simulink model "Bioreactor_for_olderversion_1_"  (R2025a)
settings: Solver=VariableStepAuto  StartTime=0.0  StopTime=2500  RelTol=1e-3
libraries: slpidlib x1, simulink x1
settings Model: Creator=a  LastModifiedBy=sayed
settings OptimizationCC: BlockReduction=off  DefaultParameterBehavior=Inlined  BufferReuse=off

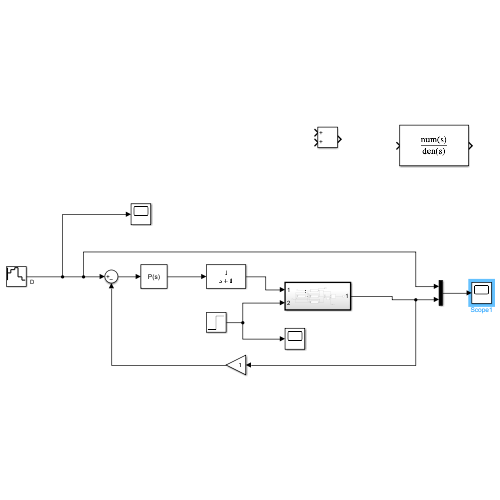
[thumbnail: Simulink's stored preview of the top-level diagram]
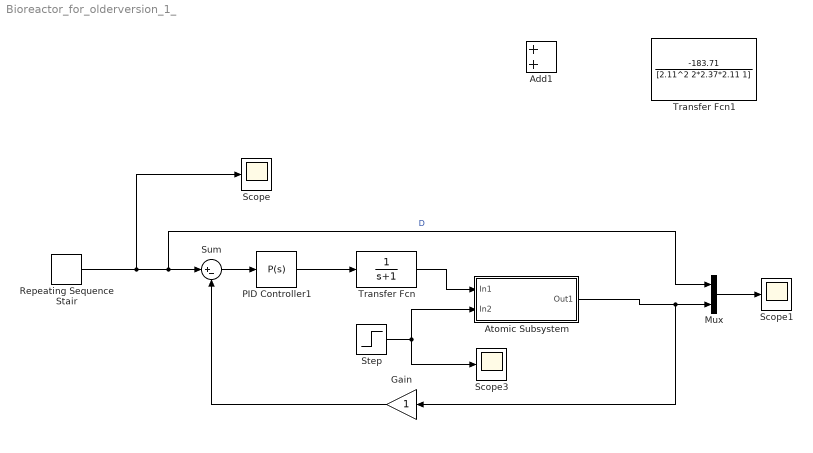
== system Bioreactor_for_olderversion_1_ ==
  Add1 : Sum
  Atomic Subsystem : Subsystem  TreatAsAtomicUnit=on
  Gain : Gain
  Mux : Mux  Inputs=2
  PID Controller1 : slpidlib/PID Controller  Controller=P  Form=Ideal  TimeDomain=Continuous-time  UseExternalTs=off  SampleTime=-1  IntegratorMethod=Forward Euler  FilterMethod=Forward Euler  ControllerParametersSource=internal  P=-0.0321  I=1/0.0992  UseKiTs=off  D=0.023  UseExternalDerivativeSource=off  N=100  UseFilter=on  TunerSelectOption=Transfer Function Based (PID Tuner App)  InitialConditionSource=internal  InitialConditionForIntegrator=0  InitialConditionForFilter=0  DifferentiatorICPrevScaledInput=0  ExternalReset=none  TrackingMode=off  Kt=1  LimitOutput=off  SatLimitsSource=internal  UpperSaturationLimit=inf  LowerSaturationLimit=-inf  LinearizeAsGain=on  AntiWindupMode=none  Kb=1  LimitIntegrator=off  UpperIntegratorSaturationLimit=inf  LowerIntegratorSaturationLimit=-inf  POutMin=[]  POutMax=[]  IOutMin=[]  IOutMax=[]  DOutMin=[]  DOutMax=[]  NOutMin=[]  NOutMax=[]  SumOutMin=[]  SumOutMax=[]  SaturationOutMin=[]  SaturationOutMax=[]  PParamMin=[]  PParamMax=[]  IParamMin=[]  IParamMax=[]  DParamMin=[]  DParamMax=[]  NParamMin=[]  NParamMax=[]  KbParamMin=[]  KbParamMax=[]  KtParamMin=[]  KtParamMax=[]  KbOutMin=[]  KbOutMax=[]  KtOutMin=[]  KtOutMax=[]  IntegratorOutMin=[]  IntegratorOutMax=[]  FilterOutMin=[]  FilterOutMax=[]  SumI1OutMin=[]  SumI1OutMax=[]  SumI2OutMin=[]  SumI2OutMax=[]  SumI3OutMin=[]  SumI3OutMax=[]  SumI4OutMin=[]  SumI4OutMax=[]  SumDOutMin=[]  SumDOutMax=[]  DifferentiatorOutMin=[]  DifferentiatorOutMax=[]  FilterDiffOutCoefMin=[]  FilterDiffOutCoefMax=[]  ReciprocalOutMin=[]  ReciprocalOutMax=[]  SumDenOutMin=[]  SumDenOutMax=[]  SumNumOutMin=[]  SumNumOutMax=[]  DivideOutMin=[]  DivideOutMax=[]  UdiffTsProdOutMin=[]  UdiffTsProdOutMax=[]  NTsProdOutMin=[]  NTsProdOutMax=[]  UintegralTsProdOutMin=[]  UintegralTsProdOutMax=[]  UngainTsProdOutMin=[]  UngainTsProdOutMax=[]  ClampingZeroOutDataTypeStr=Inherit: Inherit via back propagation  ClampingZeroOutMin=[]  ClampingZeroOutMax=[]  FilterDenConstantOutDataTypeStr=Inherit: Inherit via back propagation  FilterDenConstantOutMin=[]  FilterDenConstantOutMax=[]  PCopyOutDataTypeStr=Inherit: Inherit via back propagation  PCopyOutMin=[]  PCopyOutMax=[]  NCopyOutDataTypeStr=Inherit: Inherit via back propagation  NCopyOutMin=[]  NCopyOutMax=[]  IntegratorContinuousStateAttributes=''  IntegratorStateMustResolveToSignalObject=off  IntegratorRTWStateStorageClass=Auto  FilterContinuousStateAttributes=''  FilterStateMustResolveToSignalObject=off  FilterRTWStateStorageClass=Auto  ParallelPVariant=InternalParameters  IdealPVariant=Disabled  IVariant=Disabled  DVariant=Disabled  IntegratorVariant=Disabled  SatVariant=Disabled  AWVariant=Disabled  PCopyVariant=Disabled  TRVariant=Disabled  FdbkBlocksVariant=Forward  IdealPFdbkVariant=Disabled  SatFdbkVariant=Disabled  DerivativeFilterVariant=Disabled  NVariant=Disabled  NCopyVariant=Disabled_SignalSpec  FilterICVariant=Disabled  IntegratorICVariant=Disabled  ExternalResetVariant=Disabled  TRSumVariant=Passthrough  SumFdbkVariant=Disabled  SumVariant=Passthrough_P  TsampFilterVariant=InternalTs  TsampNgainVariant=Passthrough  TsampIntegralVariant=Disabled_SignalSpec  ExternalSaturationOutDataTypeStr=Inherit: Same as second input  DerivativeSourceVariant=Disabled  PreIntVariant=InternalPreInt
  Repeating Sequence Stair : simulink/Sources/Repeating Sequence Stair  OutValues=[2.6855 2.9 3 2.5 2.3 ].'  tsamp=500  OutMin=[]  OutMax=[]  OutDataTypeStr=double  OutputDataTypeScalingMode=double  OutDataType=fixdt(0,8)  ConRadixGroup=Best Precision: Vector-wise  OutScaling=2^-12
  Scope : Scope
      settings: ActiveDisplayYMinimum=-1  ActiveDisplayYMaximum=1
  Scope1 : Scope
      settings: ActiveDisplayYMinimum=-3.1572708705408776  ActiveDisplayYMaximum=29.415437834867905
  Scope3 : Scope
      settings: ActiveDisplayYMinimum=-1  ActiveDisplayYMaximum=1  DataLoggingVariableName=ScopeData9
  Step : Step  After=19.999  SampleTime=0
  Sum : Sum  Inputs=|+-
  Transfer Fcn : TransferFcn  Denominator=[1 1]
  Transfer Fcn1 : TransferFcn  Numerator=[-183.71]  Denominator=[2.11^2 2*2.37*2.11 1]
  wires:
  Repeating Sequence Stair/1 -> Mux/1, Sum/1, Scope/1  "D"
  Mux/1 -> Scope1/1
  Sum/1 -> PID Controller1/1
  PID Controller1/1 -> Transfer Fcn/1
  Transfer Fcn/1 -> Atomic Subsystem/1(In1)
  Gain/1 -> Sum/2
  Step/1 -> Scope3/1, Atomic Subsystem/2(In2)
  Atomic Subsystem/1(Out1) -> Gain/1, Mux/2

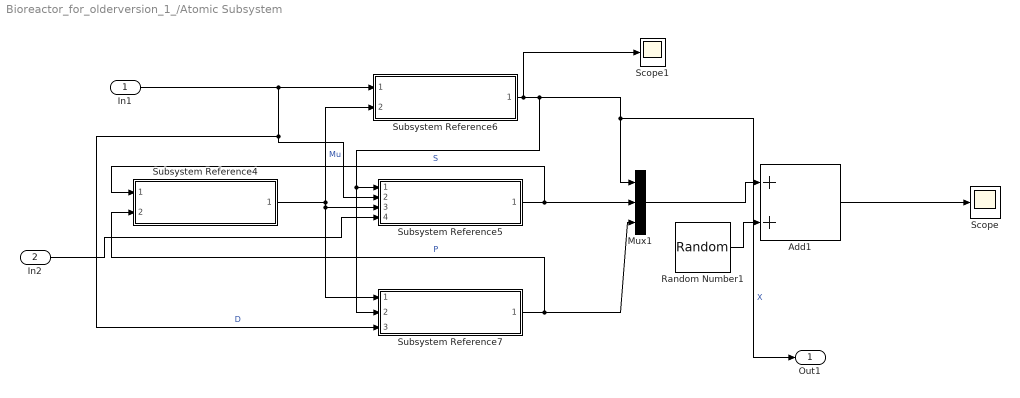
== system Bioreactor_for_olderversion_1_/Atomic Subsystem ==
  In1 : Inport
  In2 : Inport  Port=2
  Add1 : Sum
  Mux1 : Mux  Inputs=3
  Random Number1 : RandomNumber  Variance=0.01  SampleTime=0.1
  Scope : Scope
      settings: ActiveDisplayYMinimum=-9798.9196176080059  ActiveDisplayYMaximum=28688.615167165182  DataLoggingVariableName=ScopeData6
  Scope1 : Scope
      settings: ActiveDisplayYMinimum=-1  ActiveDisplayYMaximum=1  DataLoggingVariableName=ScopeData7
  Subsystem Reference4 : Subsystem  ReferencedSubsystem=Mu_SP_oldversion
  Subsystem Reference5 : Subsystem  ReferencedSubsystem=Substrate_oldVersion
  Subsystem Reference6 : Subsystem  ReferencedSubsystem=Biomass_X_oldversion
  Subsystem Reference7 : Subsystem  ReferencedSubsystem=Product_P_oldversion
  Out1 : Outport
  wires:
  Subsystem Reference6/1 -> Scope1/1, Out1/1, Mux1/1, Subsystem Reference7/2, Subsystem Reference5/1  "X"
  Random Number1/1 -> Add1/2
  Subsystem Reference7/1 -> Subsystem Reference4/2, Mux1/3  "P"
  Mux1/1 -> Add1/1
  Subsystem Reference5/1 -> Mux1/2, Subsystem Reference4/1  "S"
  Subsystem Reference4/1 -> Subsystem Reference7/1, Subsystem Reference5/3, Subsystem Reference6/2  "Mu"
  Add1/1 -> Scope/1
  In1/1 -> Subsystem Reference7/3, Subsystem Reference5/2, Subsystem Reference6/1  "D"
  In2/1 -> Subsystem Reference5/4
